simulink model "e4_tank_reactor_no_error_dyn"  (R2020a)
settings: Solver=FixedStepAuto  StartTime=0.0  StopTime=options.T_train  FixedStep=options.dt  RelTol=1e-3
PreLoadFcn:
  | load e4_PIDGainSchedExample.mat
model workspace (MAT data in the model file):
  op_snapshot1 : handle (value not decoded)
values from neighbouring files (symbols this model uses):
  C = [2 3 4 5 6 7 8 9]    [e4_PIDGainSchedExample.mat]
undefined symbols (not defined in the file or in its folder): Controllers, D, I, N, options, P, sigbuilder_block
libraries: neural x132, simulink x2, simulink_need_slupdate x1
(part 4 of 6)

== system e4_tank_reactor_no_error_dyn/NN/Layer 3/Delays 1 ==
  "p{3}" : Inport  PortDimensions=30
      mask Display: e = 0.06;c1 = [120 230 180]/255;c2 = ([120 230 180]+0)/(256+128);c3 = ([120 230 180]+128)/(256+128);patch([0 1 1 0],[0 0 1 1],c1);patch([0 1 1 1-e 1-e 0+e],[0 0 1 1-e 0+e 0+e],c2);patch([0 0 1 1-e 0+e 0+e],[0 1 1 1-e 1-e 0+e],c3);plot([0 1 1 0 0],[0 0 1 1 0]);
  mux : Mux  Inputs=1
      mask Display: e = 0.06;c1 = [120 150 230]/255;c2 = ([120 150 230]+0)/383;c3 = ([120 150 230]+128)/383;patch([0 1 1 0],[0 0 1 1],c1);patch([0 1 1 1-e 1-e 0+e],[0 0 1 1-e 0+e 0+e],c2);patch([0 0 1 1-e 0+e 0+e],[0 1 1 1-e 1-e 0+e],c3);plot([0 1 1 0 0],[0 0 1 1 0]);disp('Mux')
  "pd{3,2}" : Outport
      mask Display: e = 0.06;c1 = [120 230 180]/255;c2 = ([120 230 180]+0)/(256+128);c3 = ([120 230 180]+128)/(256+128);patch([0 1 1 0],[0 0 1 1],c1);patch([0 1 1 1-e 1-e 0+e],[0 0 1 1-e 0+e 0+e],c2);patch([0 0 1 1-e 0+e 0+e],[0 1 1 1-e 1-e 0+e],c3);plot([0 1 1 0 0],[0 0 1 1 0]);
  wires:
  "p{3}"/1 -> mux/1
  mux/1 -> "pd{3,2}"/1

== system e4_tank_reactor_no_error_dyn/NN/Layer 3/LW{3,2} ==
  "ad{3,2}" : Inport  PortDimensions=30
      mask Display: e = 0.06;c1 = [120 230 180]/255;c2 = ([120 230 180]+0)/(256+128);c3 = ([120 230 180]+128)/(256+128);patch([0 1 1 0],[0 0 1 1],c1);patch([0 1 1 1-e 1-e 0+e],[0 0 1 1-e 0+e 0+e],c2);patch([0 0 1 1-e 0+e 0+e],[0 1 1 1-e 1-e 0+e],c3);plot([0 1 1 0 0],[0 0 1 1 0]);
  "IW{3,2}(1,:)'" : Constant  Value=[-0.0464803788192958700076218292451812885701656341552734375;-0.22366786030205820789973358841962181031703948974609375;0.09453253511773705708431947414283058606088161468505859375;0.303300315972412859455431544120074249804019927978515625;-0.001379384046064999029546083164632364059798419475555419921875;-0.11257074515520755497721694382562418468296527862548828125;-0.10240733375565913565452547118184156715869903564453125;0.05926219251905744112018936675667646341025829315185546875;-0.1213117218938437880115799316627089865505695343017578125;-0.07223384242120071963011440629998105578124523162841796875;-0.08011048819587056335489450020759250037372112274169921875;-0.01346694101269302508427916365008059074170887470245361328125;-0.0161980791466645283882552774912255699746310710906982421875;-0.13100020285189517554869098603376187384128570556640625;-0.325236116042997736030883970670402050018310546875;-0.016627521139407630546003247218322940170764923095703125;0.01071971917916101670054107586338432156480848789215087890625;-0.00444701838994284413819624290908905095420777797698974609375;0.066701814396379177640739044363726861774921417236328125;0.097044878239975762568292338983155786991119384765625;-0.24982480627273417894684826023876667022705078125;-0.0259297241783282804428178991429376765154302120208740234375;0.176353365166070863434555349158472381532192230224609375;-0.0778415585458839542898346053334535099565982818603515625;0.28946783805742037909425334873958490788936614990234375;-0.0264164360665425819452156730449132737703621387481689453125;0.039973819515048851502836413374097901396453380584716796875;0.08025452129389230859768389336750260554254055023193359375;0.4427935738953550082186438885401003062725067138671875;-0.344840403191533029225723794297664426267147064208984375]
      mask Display: e = 0.06;c1 = [120 150 230]/255;c2 = ([120 150 230]+0)/383;c3 = ([120 150 230]+128)/383;patch([0 1 1 0],[0 0 1 1],c1);patch([0 1 1 1-e 1-e 0+e],[0 0 1 1-e 0+e 0+e],c2);patch([0 0 1 1-e 0+e 0+e],[0 1 1 1-e 1-e 0+e],c3);plot([0 1 1 0 0],[0 0 1 1 0]);disp('weights');
  Mux : Mux  Inputs=1
      mask Display: e = 0.06;c1 = [120 150 230]/255;c2 = ([120 150 230]+0)/383;c3 = ([120 150 230]+128)/383;patch([0 1 1 0],[0 0 1 1],c1);patch([0 1 1 1-e 1-e 0+e],[0 0 1 1-e 0+e 0+e],c2);patch([0 0 1 1-e 0+e 0+e],[0 1 1 1-e 1-e 0+e],c3);plot([0 1 1 0 0],[0 0 1 1 0]);disp('Mux');
  dotprod1 : neural/Weight Functions/dotprod
  "lz{3,2}" : Outport
      mask Display: e = 0.06;c1 = [120 230 180]/255;c2 = ([120 230 180]+0)/(256+128);c3 = ([120 230 180]+128)/(256+128);patch([0 1 1 0],[0 0 1 1],c1);patch([0 1 1 1-e 1-e 0+e],[0 0 1 1-e 0+e 0+e],c2);patch([0 0 1 1-e 0+e 0+e],[0 1 1 1-e 1-e 0+e],c3);plot([0 1 1 0 0],[0 0 1 1 0]);
  wires:
  "IW{3,2}(1,:)'"/1 -> dotprod1/1
  "ad{3,2}"/1 -> dotprod1/2
  dotprod1/1 -> Mux/1
  Mux/1 -> "lz{3,2}"/1

== system e4_tank_reactor_no_error_dyn/NN_cex_1/Layer 1/Delays 1 ==
  "p{1}" : Inport  PortDimensions=8
      mask Display: e = 0.06;c1 = [120 230 180]/255;c2 = ([120 230 180]+0)/(256+128);c3 = ([120 230 180]+128)/(256+128);patch([0 1 1 0],[0 0 1 1],c1);patch([0 1 1 1-e 1-e 0+e],[0 0 1 1-e 0+e 0+e],c2);patch([0 0 1 1-e 0+e 0+e],[0 1 1 1-e 1-e 0+e],c3);plot([0 1 1 0 0],[0 0 1 1 0]);
  mux : Mux  Inputs=1
      mask Display: e = 0.06;c1 = [120 150 230]/255;c2 = ([120 150 230]+0)/383;c3 = ([120 150 230]+128)/383;patch([0 1 1 0],[0 0 1 1],c1);patch([0 1 1 1-e 1-e 0+e],[0 0 1 1-e 0+e 0+e],c2);patch([0 0 1 1-e 0+e 0+e],[0 1 1 1-e 1-e 0+e],c3);plot([0 1 1 0 0],[0 0 1 1 0]);disp('Mux')
  "pd{1,1}" : Outport
      mask Display: e = 0.06;c1 = [120 230 180]/255;c2 = ([120 230 180]+0)/(256+128);c3 = ([120 230 180]+128)/(256+128);patch([0 1 1 0],[0 0 1 1],c1);patch([0 1 1 1-e 1-e 0+e],[0 0 1 1-e 0+e 0+e],c2);patch([0 0 1 1-e 0+e 0+e],[0 1 1 1-e 1-e 0+e],c3);plot([0 1 1 0 0],[0 0 1 1 0]);
  wires:
  "p{1}"/1 -> mux/1
  mux/1 -> "pd{1,1}"/1

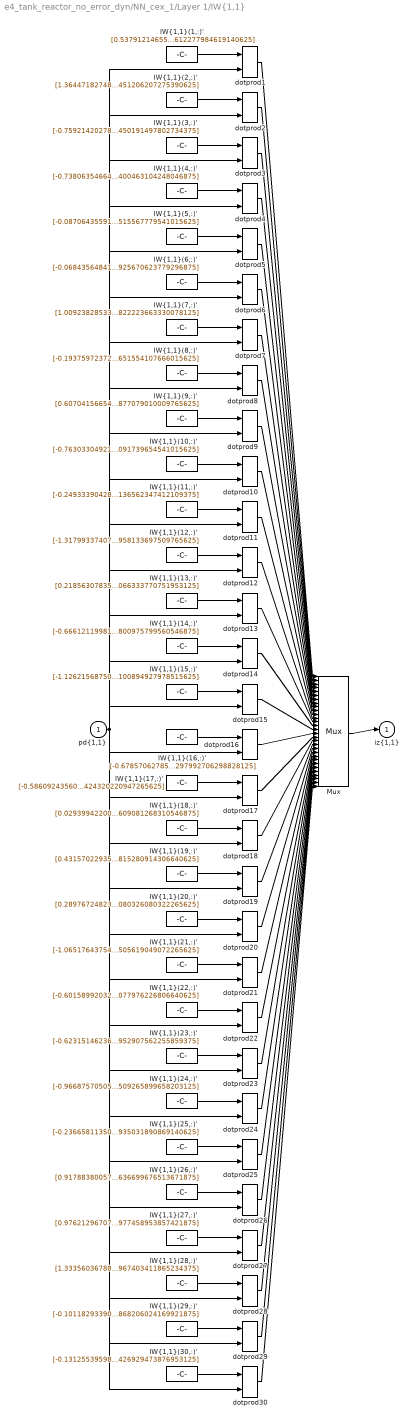
== system e4_tank_reactor_no_error_dyn/NN_cex_1/Layer 1/IW{1,1} ==
  "pd{1,1}" : Inport  PortDimensions=8
      mask Display: e = 0.06;c1 = [120 230 180]/255;c2 = ([120 230 180]+0)/(256+128);c3 = ([120 230 180]+128)/(256+128);patch([0 1 1 0],[0 0 1 1],c1);patch([0 1 1 1-e 1-e 0+e],[0 0 1 1-e 0+e 0+e],c2);patch([0 0 1 1-e 0+e 0+e],[0 1 1 1-e 1-e 0+e],c3);plot([0 1 1 0 0],[0 0 1 1 0]);
  "IW{1,1}(1,:)'" : Constant  Value=[0.5379121465548728497907404744182713329792022705078125;-0.4891956453284975747664020673255436122417449951171875;0.453842574705631829345975347678177058696746826171875;-2.25657579421494514093637917540036141872406005859375;-0.2491786341732944720650522185678710229694843292236328125;-0.1742315599251909319367115358545561321079730987548828125;-1.8134520137386844762517057461082004010677337646484375;-0.86465480796345206560005181017913855612277984619140625]
      mask Display: e = 0.06;c1 = [120 150 230]/255;c2 = ([120 150 230]+0)/383;c3 = ([120 150 230]+128)/383;patch([0 1 1 0],[0 0 1 1],c1);patch([0 1 1 1-e 1-e 0+e],[0 0 1 1-e 0+e 0+e],c2);patch([0 0 1 1-e 0+e 0+e],[0 1 1 1-e 1-e 0+e],c3);plot([0 1 1 0 0],[0 0 1 1 0]);disp('Weights');
  "IW{1,1}(10,:)'" : Constant  Value=[-0.7630330492125356744992359381285496056079864501953125;-0.1535957203894409150990441048634238541126251220703125;-1.1348681599380225915041364714852534234523773193359375;1.1072262797523821920009368113824166357517242431640625;-0.5333903505207240325347584075643680989742279052734375;-0.51407599439698958843081300074118189513683319091796875;1.1142771208274837579921268115867860615253448486328125;-1.5225707798856602526171855060965754091739654541015625]
      mask Display: e = 0.06;c1 = [120 150 230]/255;c2 = ([120 150 230]+0)/383;c3 = ([120 150 230]+128)/383;patch([0 1 1 0],[0 0 1 1],c1);patch([0 1 1 1-e 1-e 0+e],[0 0 1 1-e 0+e 0+e],c2);patch([0 0 1 1-e 0+e 0+e],[0 1 1 1-e 1-e 0+e],c3);plot([0 1 1 0 0],[0 0 1 1 0]);disp('Weights');
  "IW{1,1}(11,:)'" : Constant  Value=[-0.2493339042877996403202445208080462180078029632568359375;-0.044937110292640324027413356589022441767156124114990234375;-0.89629168879976617301252872493932954967021942138671875;-0.94562916108070871334945195485488511621952056884765625;1.1876936211677457944091429453692398965358734130859375;-0.54144662550112754306752549382508732378482818603515625;1.0278469665745559868952341275871731340885162353515625;-0.47008241850572252129580874679959379136562347412109375]
      mask Display: e = 0.06;c1 = [120 150 230]/255;c2 = ([120 150 230]+0)/383;c3 = ([120 150 230]+128)/383;patch([0 1 1 0],[0 0 1 1],c1);patch([0 1 1 1-e 1-e 0+e],[0 0 1 1-e 0+e 0+e],c2);patch([0 0 1 1-e 0+e 0+e],[0 1 1 1-e 1-e 0+e],c3);plot([0 1 1 0 0],[0 0 1 1 0]);disp('Weights');
  "IW{1,1}(12,:)'" : Constant  Value=[-1.31799337407540662070459802635014057159423828125;1.08939525062658759679834474809467792510986328125;1.100424298584484983365427979151718318462371826171875;-0.35666979575481694286764877688256092369556427001953125;0.293602012746428442380164369751582853496074676513671875;0.98047102923849960287583371609798632562160491943359375;-0.4527363536410680122656913226819597184658050537109375;0.78261151530452244262647809591726399958133697509765625]
      mask Display: e = 0.06;c1 = [120 150 230]/255;c2 = ([120 150 230]+0)/383;c3 = ([120 150 230]+128)/383;patch([0 1 1 0],[0 0 1 1],c1);patch([0 1 1 1-e 1-e 0+e],[0 0 1 1-e 0+e 0+e],c2);patch([0 0 1 1-e 0+e 0+e],[0 1 1 1-e 1-e 0+e],c3);plot([0 1 1 0 0],[0 0 1 1 0]);disp('Weights');
  "IW{1,1}(13,:)'" : Constant  Value=[0.2185630783525124576360809669495210982859134674072265625;1.153492150410983629882366585661657154560089111328125;-0.281741742390723970412835797105799429118633270263671875;0.430450607409247065771040752224507741630077362060546875;-0.2156642293311239744202367774050799198448657989501953125;-1.28844042664953928323257059673778712749481201171875;0.226045890241030555944945490409736521542072296142578125;0.81490911166711743618407126632519066333770751953125]
      mask Display: e = 0.06;c1 = [120 150 230]/255;c2 = ([120 150 230]+0)/383;c3 = ([120 150 230]+128)/383;patch([0 1 1 0],[0 0 1 1],c1);patch([0 1 1 1-e 1-e 0+e],[0 0 1 1-e 0+e 0+e],c2);patch([0 0 1 1-e 0+e 0+e],[0 1 1 1-e 1-e 0+e],c3);plot([0 1 1 0 0],[0 0 1 1 0]);disp('Weights');
  "IW{1,1}(14,:)'" : Constant  Value=[-0.66612119981264938939347075574914924800395965576171875;0.70433163322524794391910063495743088424205780029296875;1.51350451798926766144859357154928147792816162109375;0.135062226669892371244685591591405682265758514404296875;-0.6139892191890223838157680802396498620510101318359375;0.785352351475125498581064675818197429180145263671875;0.2797159376970330679768039772170595824718475341796875;2.02825949533217197995327296666800975799560546875]
      mask Display: e = 0.06;c1 = [120 150 230]/255;c2 = ([120 150 230]+0)/383;c3 = ([120 150 230]+128)/383;patch([0 1 1 0],[0 0 1 1],c1);patch([0 1 1 1-e 1-e 0+e],[0 0 1 1-e 0+e 0+e],c2);patch([0 0 1 1-e 0+e 0+e],[0 1 1 1-e 1-e 0+e],c3);plot([0 1 1 0 0],[0 0 1 1 0]);disp('Weights');
  "IW{1,1}(15,:)'" : Constant  Value=[-1.126215687500734308201799649395979940891265869140625;0.5324020585546609396487838239409029483795166015625;0.275269474209976883205541753341094590723514556884765625;0.9901222314779591915367973342654295265674591064453125;-0.8749086639717464919385747634805738925933837890625;0.38958898768835348302985721602453850209712982177734375;-0.073311773987459749601924841044819913804531097412109375;0.84648532346684801641600870425463654100894927978515625]
      mask Display: e = 0.06;c1 = [120 150 230]/255;c2 = ([120 150 230]+0)/383;c3 = ([120 150 230]+128)/383;patch([0 1 1 0],[0 0 1 1],c1);patch([0 1 1 1-e 1-e 0+e],[0 0 1 1-e 0+e 0+e],c2);patch([0 0 1 1-e 0+e 0+e],[0 1 1 1-e 1-e 0+e],c3);plot([0 1 1 0 0],[0 0 1 1 0]);disp('Weights');
  "IW{1,1}(16,:)'" : Constant  Value=[-0.6785706278511709488299175063730217516422271728515625;-1.1815839277690927122677067018230445683002471923828125;-0.70641636384911199453284780247486196458339691162109375;1.0070190226252275778051625820808112621307373046875;0.0220071147234353892141456299214041791856288909912109375;0.0942288635999547763422157231616438366472721099853515625;0.9300673100145997462817604173324070870876312255859375;1.23984567310700288800262569566257297992706298828125]
      mask Display: e = 0.06;c1 = [120 150 230]/255;c2 = ([120 150 230]+0)/383;c3 = ([120 150 230]+128)/383;patch([0 1 1 0],[0 0 1 1],c1);patch([0 1 1 1-e 1-e 0+e],[0 0 1 1-e 0+e 0+e],c2);patch([0 0 1 1-e 0+e 0+e],[0 1 1 1-e 1-e 0+e],c3);plot([0 1 1 0 0],[0 0 1 1 0]);disp('Weights');
  "IW{1,1}(17,:)'" : Constant  Value=[-0.5860924356005476898445749611710198223590850830078125;0.851474377071834709340691915713250637054443359375;-0.1567050173144934610558465237772907130420207977294921875;-0.68500297234766527321170315190101973712444305419921875;0.8118387502084571938354429221362806856632232666015625;-1.154822097518132917315369923016987740993499755859375;0.60957063637892872076662342806230299174785614013671875;0.375224662295090161112653959207818843424320220947265625]
      mask Display: e = 0.06;c1 = [120 150 230]/255;c2 = ([120 150 230]+0)/383;c3 = ([120 150 230]+128)/383;patch([0 1 1 0],[0 0 1 1],c1);patch([0 1 1 1-e 1-e 0+e],[0 0 1 1-e 0+e 0+e],c2);patch([0 0 1 1-e 0+e 0+e],[0 1 1 1-e 1-e 0+e],c3);plot([0 1 1 0 0],[0 0 1 1 0]);disp('Weights');
  "IW{1,1}(18,:)'" : Constant  Value=[0.02939942200266887351034483799594454467296600341796875;-0.299792566816287131548079969434184022247791290283203125;-0.60369148945598005706614230803097598254680633544921875;-0.13551079379416908210487235919572412967681884765625;0.419757903271528010069602032672264613211154937744140625;0.799628628682101716407260028063319623470306396484375;0.5142029788862163552920492293196730315685272216796875;-0.223354218656821312816163072056951932609081268310546875]
      mask Display: e = 0.06;c1 = [120 150 230]/255;c2 = ([120 150 230]+0)/383;c3 = ([120 150 230]+128)/383;patch([0 1 1 0],[0 0 1 1],c1);patch([0 1 1 1-e 1-e 0+e],[0 0 1 1-e 0+e 0+e],c2);patch([0 0 1 1-e 0+e 0+e],[0 1 1 1-e 1-e 0+e],c3);plot([0 1 1 0 0],[0 0 1 1 0]);disp('Weights');
  "IW{1,1}(19,:)'" : Constant  Value=[0.431570229354902357155054914983338676393032073974609375;0.3345690055866470391521261262823827564716339111328125;1.0469583717854737958674604669795371592044830322265625;0.72253391100106190148011364726698957383632659912109375;-0.545424201225733984443877488956786692142486572265625;0.0101024782301144915030999271721157128922641277313232421875;-0.167124150696403350746521709879743866622447967529296875;-1.454795311551409842110160752781666815280914306640625]
      mask Display: e = 0.06;c1 = [120 150 230]/255;c2 = ([120 150 230]+0)/383;c3 = ([120 150 230]+128)/383;patch([0 1 1 0],[0 0 1 1],c1);patch([0 1 1 1-e 1-e 0+e],[0 0 1 1-e 0+e 0+e],c2);patch([0 0 1 1-e 0+e 0+e],[0 1 1 1-e 1-e 0+e],c3);plot([0 1 1 0 0],[0 0 1 1 0]);disp('Weights');
  "IW{1,1}(2,:)'" : Constant  Value=[1.3644718274849083616828693266143091022968292236328125;-0.6113012571242200099419505932019092142581939697265625;0.219308348802042252234656416476354934275150299072265625;-0.050551389902864729553044753629365004599094390869140625;1.1572125475706760422411889521754346787929534912109375;0.364957647871666068795093451626598834991455078125;1.3711534269785918827011528264847584068775177001953125;-0.634282382592994853354184670024551451206207275390625]
      mask Display: e = 0.06;c1 = [120 150 230]/255;c2 = ([120 150 230]+0)/383;c3 = ([120 150 230]+128)/383;patch([0 1 1 0],[0 0 1 1],c1);patch([0 1 1 1-e 1-e 0+e],[0 0 1 1-e 0+e 0+e],c2);patch([0 0 1 1-e 0+e 0+e],[0 1 1 1-e 1-e 0+e],c3);plot([0 1 1 0 0],[0 0 1 1 0]);disp('Weights');
  "IW{1,1}(20,:)'" : Constant  Value=[0.289767248236110164238965580807416699826717376708984375;-1.6550121300658424683405200994457118213176727294921875;0.66498678015265133556255250368849374353885650634765625;-0.358201489276206597178742185860755853354930877685546875;1.2038940893287257694055369938723742961883544921875;-0.7811727388937643734578841758775524795055389404296875;-0.293491754609760124861139729546266607940196990966796875;-0.87310715343854161663017521277652122080326080322265625]
      mask Display: e = 0.06;c1 = [120 150 230]/255;c2 = ([120 150 230]+0)/383;c3 = ([120 150 230]+128)/383;patch([0 1 1 0],[0 0 1 1],c1);patch([0 1 1 1-e 1-e 0+e],[0 0 1 1-e 0+e 0+e],c2);patch([0 0 1 1-e 0+e 0+e],[0 1 1 1-e 1-e 0+e],c3);plot([0 1 1 0 0],[0 0 1 1 0]);disp('Weights');
  "IW{1,1}(21,:)'" : Constant  Value=[-1.0651764375415757601928135045454837381839752197265625;-0.05093105960695791523118458599128643982112407684326171875;0.10166969326193157907578523690972360782325267791748046875;0.787265018557109730323873009183444082736968994140625;-1.0383486929548138011369928790372796356678009033203125;1.0418870137961391275638334263931028544902801513671875;-2.059969041537390577190080875880084931850433349609375;-0.363346918231178594993480146513320505619049072265625]
      mask Display: e = 0.06;c1 = [120 150 230]/255;c2 = ([120 150 230]+0)/383;c3 = ([120 150 230]+128)/383;patch([0 1 1 0],[0 0 1 1],c1);patch([0 1 1 1-e 1-e 0+e],[0 0 1 1-e 0+e 0+e],c2);patch([0 0 1 1-e 0+e 0+e],[0 1 1 1-e 1-e 0+e],c3);plot([0 1 1 0 0],[0 0 1 1 0]);disp('Weights');
  "IW{1,1}(22,:)'" : Constant  Value=[-0.60158992032533775695668509797542355954647064208984375;-1.3680290127964724877784874479402787983417510986328125;-0.87834865591767175008186541163013316690921783447265625;-0.2207869194855082983774963167888927273452281951904296875;-0.11766408992345871176166127725082333199679851531982421875;0.97286536737283990650126952459686435759067535400390625;-0.76589398294444854808915579269523732364177703857421875;-0.449268913356635213318668320425786077976226806640625]
      mask Display: e = 0.06;c1 = [120 150 230]/255;c2 = ([120 150 230]+0)/383;c3 = ([120 150 230]+128)/383;patch([0 1 1 0],[0 0 1 1],c1);patch([0 1 1 1-e 1-e 0+e],[0 0 1 1-e 0+e 0+e],c2);patch([0 0 1 1-e 0+e 0+e],[0 1 1 1-e 1-e 0+e],c3);plot([0 1 1 0 0],[0 0 1 1 0]);disp('Weights');
  "IW{1,1}(23,:)'" : Constant  Value=[-0.62315146236465379647739837309927679598331451416015625;0.700611887631571672585550913936458528041839599609375;-1.253865587185787777713130708434619009494781494140625;0.12191954613290224840316255949801416136324405670166015625;0.02485690435094556338668780881562270224094390869140625;-0.97564300724903951778088639912311919033527374267578125;-1.3728328336670490017468182486481964588165283203125;-0.476364886346988425369630704153678379952907562255859375]
      mask Display: e = 0.06;c1 = [120 150 230]/255;c2 = ([120 150 230]+0)/383;c3 = ([120 150 230]+128)/383;patch([0 1 1 0],[0 0 1 1],c1);patch([0 1 1 1-e 1-e 0+e],[0 0 1 1-e 0+e 0+e],c2);patch([0 0 1 1-e 0+e 0+e],[0 1 1 1-e 1-e 0+e],c3);plot([0 1 1 0 0],[0 0 1 1 0]);disp('Weights');
  "IW{1,1}(24,:)'" : Constant  Value=[-0.9668757050519467544091867239330895245075225830078125;1.8074949802424502554032414991525001823902130126953125;0.1509264792134751009822224432355142198503017425537109375;0.56079147047206401310859291697852313518524169921875;-0.86686870292866513576512943473062478005886077880859375;0.00566384031475077563688724779922267771326005458831787109375;-0.5858846977314049464524714494473300874233245849609375;-0.35202968611922369479572125783306546509265899658203125]
      mask Display: e = 0.06;c1 = [120 150 230]/255;c2 = ([120 150 230]+0)/383;c3 = ([120 150 230]+128)/383;patch([0 1 1 0],[0 0 1 1],c1);patch([0 1 1 1-e 1-e 0+e],[0 0 1 1-e 0+e 0+e],c2);patch([0 0 1 1-e 0+e 0+e],[0 1 1 1-e 1-e 0+e],c3);plot([0 1 1 0 0],[0 0 1 1 0]);disp('Weights');
  "IW{1,1}(25,:)'" : Constant  Value=[-0.2366581135092546139819802419879124499857425689697265625;-1.1565509789181909194866193502093665301799774169921875;0.356085223857672328318102472621831111609935760498046875;0.51409424697715355723204311289009638130664825439453125;-0.73596497723560927450847657382837496697902679443359375;0.2926871688236143409511669233324937522411346435546875;-1.3190253126527398119804956877487711608409881591796875;1.3400461156173195664820241290726698935031890869140625]
      mask Display: e = 0.06;c1 = [120 150 230]/255;c2 = ([120 150 230]+0)/383;c3 = ([120 150 230]+128)/383;patch([0 1 1 0],[0 0 1 1],c1);patch([0 1 1 1-e 1-e 0+e],[0 0 1 1-e 0+e 0+e],c2);patch([0 0 1 1-e 0+e 0+e],[0 1 1 1-e 1-e 0+e],c3);plot([0 1 1 0 0],[0 0 1 1 0]);disp('Weights');
  "IW{1,1}(26,:)'" : Constant  Value=[0.91788380057172869186388197704218327999114990234375;1.15538220933264046408339709159918129444122314453125;0.8339026184910924843762813907233066856861114501953125;0.36652474061263762283857658985652960836887359619140625;-0.038492407008773772691956338576346752233803272247314453125;0.10236621810067032811719656137938727624714374542236328125;0.6540196398808897360055425451719202101230621337890625;0.3290186601830498158705040623317472636699676513671875]
      mask Display: e = 0.06;c1 = [120 150 230]/255;c2 = ([120 150 230]+0)/383;c3 = ([120 150 230]+128)/383;patch([0 1 1 0],[0 0 1 1],c1);patch([0 1 1 1-e 1-e 0+e],[0 0 1 1-e 0+e 0+e],c2);patch([0 0 1 1-e 0+e 0+e],[0 1 1 1-e 1-e 0+e],c3);plot([0 1 1 0 0],[0 0 1 1 0]);disp('Weights');
  "IW{1,1}(27,:)'" : Constant  Value=[0.9762129670729109420790337026119232177734375;-0.66682266891450880930136690949439071118831634521484375;0.14765647832353767654467446845956146717071533203125;-0.744789681230276556789249298162758350372314453125;0.664196844738051073164797344361431896686553955078125;0.74611195556748632906618468041415326297283172607421875;0.796280949331405363267322172760032117366790771484375;-0.1026615824494294393343096771786804310977458953857421875]
      mask Display: e = 0.06;c1 = [120 150 230]/255;c2 = ([120 150 230]+0)/383;c3 = ([120 150 230]+128)/383;patch([0 1 1 0],[0 0 1 1],c1);patch([0 1 1 1-e 1-e 0+e],[0 0 1 1-e 0+e 0+e],c2);patch([0 0 1 1-e 0+e 0+e],[0 1 1 1-e 1-e 0+e],c3);plot([0 1 1 0 0],[0 0 1 1 0]);disp('Weights');
  "IW{1,1}(28,:)'" : Constant  Value=[1.33356036788779430679596771369688212871551513671875;0.2356965321398985790946056795291951857507228851318359375;-0.232455208957773551414760504485457204282283782958984375;-0.178559020015909786227581435014144517481327056884765625;0.89276443639134417384894959468510933220386505126953125;-0.7558328227887614048086106777191162109375;0.1388690330901915237493682298008934594690799713134765625;1.4965266154135272724801097865565679967403411865234375]
      mask Display: e = 0.06;c1 = [120 150 230]/255;c2 = ([120 150 230]+0)/383;c3 = ([120 150 230]+128)/383;patch([0 1 1 0],[0 0 1 1],c1);patch([0 1 1 1-e 1-e 0+e],[0 0 1 1-e 0+e 0+e],c2);patch([0 0 1 1-e 0+e 0+e],[0 1 1 1-e 1-e 0+e],c3);plot([0 1 1 0 0],[0 0 1 1 0]);disp('Weights');
  "IW{1,1}(29,:)'" : Constant  Value=[-0.10118293390951231536245558118025655858218669891357421875;0.06434138355125963715241965701352455653250217437744140625;-0.69739459415743121351027866694494150578975677490234375;0.79226095210926195111511560753569938242435455322265625;-0.90436354784671169060317197363474406301975250244140625;-1.23209955543295990310070919804275035858154296875;1.092697805682678602323676386731676757335662841796875;0.4849451497525627541307358114863745868206024169921875]
      mask Display: e = 0.06;c1 = [120 150 230]/255;c2 = ([120 150 230]+0)/383;c3 = ([120 150 230]+128)/383;patch([0 1 1 0],[0 0 1 1],c1);patch([0 1 1 1-e 1-e 0+e],[0 0 1 1-e 0+e 0+e],c2);patch([0 0 1 1-e 0+e 0+e],[0 1 1 1-e 1-e 0+e],c3);plot([0 1 1 0 0],[0 0 1 1 0]);disp('Weights');
  "IW{1,1}(3,:)'" : Constant  Value=[-0.75921420278456952512868838311987929046154022216796875;1.1246289809493703604204029034008271992206573486328125;0.357400133672493292014138432932668365538120269775390625;-1.2713477569867224215016676680534146726131439208984375;0.79391674854068738920176429019193165004253387451171875;0.71648590916453891441761925307218916714191436767578125;0.359501923755549401828801592273521237075328826904296875;0.44836330481205288744916970244958065450191497802734375]
      mask Display: e = 0.06;c1 = [120 150 230]/255;c2 = ([120 150 230]+0)/383;c3 = ([120 150 230]+128)/383;patch([0 1 1 0],[0 0 1 1],c1);patch([0 1 1 1-e 1-e 0+e],[0 0 1 1-e 0+e 0+e],c2);patch([0 0 1 1-e 0+e 0+e],[0 1 1 1-e 1-e 0+e],c3);plot([0 1 1 0 0],[0 0 1 1 0]);disp('Weights');
  "IW{1,1}(30,:)'" : Constant  Value=[-0.13125539598877633551410326617769896984100341796875;-1.369496947258934227420468232594430446624755859375;-1.236078110166821009130444508627988398075103759765625;-0.72204748831942466846811612413148395717144012451171875;0.761983709141599963032831510645337402820587158203125;0.90521509240511310867560723636415787041187286376953125;-0.610208060498799387261215088074095547199249267578125;-0.78955110194053024219584813181427307426929473876953125]
      mask Display: e = 0.06;c1 = [120 150 230]/255;c2 = ([120 150 230]+0)/383;c3 = ([120 150 230]+128)/383;patch([0 1 1 0],[0 0 1 1],c1);patch([0 1 1 1-e 1-e 0+e],[0 0 1 1-e 0+e 0+e],c2);patch([0 0 1 1-e 0+e 0+e],[0 1 1 1-e 1-e 0+e],c3);plot([0 1 1 0 0],[0 0 1 1 0]);disp('Weights');
  "IW{1,1}(4,:)'" : Constant  Value=[-0.73806354664510143148703491533524356782436370849609375;-1.685791217549649001483658139477483928203582763671875;0.34882725222296262490573326431331224739551544189453125;-0.736035017934379087733987034880556166172027587890625;0.44053466594436374581533755190321244299411773681640625;0.412365071467659161097429887377074919641017913818359375;-0.2378886841219116921042342482905951328575611114501953125;0.7315009545194779416732444587978534400463104248046875]
      mask Display: e = 0.06;c1 = [120 150 230]/255;c2 = ([120 150 230]+0)/383;c3 = ([120 150 230]+128)/383;patch([0 1 1 0],[0 0 1 1],c1);patch([0 1 1 1-e 1-e 0+e],[0 0 1 1-e 0+e 0+e],c2);patch([0 0 1 1-e 0+e 0+e],[0 1 1 1-e 1-e 0+e],c3);plot([0 1 1 0 0],[0 0 1 1 0]);disp('Weights');
  "IW{1,1}(5,:)'" : Constant  Value=[-0.087064355913521851437764098591287620365619659423828125;-0.69226769568504764595928691051085479557514190673828125;-0.052166682908634430526628733559846295975148677825927734375;-1.78817229179241365955022047273814678192138671875;-0.202354836069230825668086026780656538903713226318359375;0.424849282091239732750409530126489698886871337890625;0.135767011506318480140720339477411471307277679443359375;0.80800721671806796653214632897288538515567779541015625]
      mask Display: e = 0.06;c1 = [120 150 230]/255;c2 = ([120 150 230]+0)/383;c3 = ([120 150 230]+128)/383;patch([0 1 1 0],[0 0 1 1],c1);patch([0 1 1 1-e 1-e 0+e],[0 0 1 1-e 0+e 0+e],c2);patch([0 0 1 1-e 0+e 0+e],[0 1 1 1-e 1-e 0+e],c3);plot([0 1 1 0 0],[0 0 1 1 0]);disp('Weights');
  "IW{1,1}(6,:)'" : Constant  Value=[-0.068435648417951522315405554763856343924999237060546875;0.470302497384609774488950506565743125975131988525390625;-0.94847648407455376062813456883304752409458160400390625;-0.726406908026099973341160875861532986164093017578125;-1.0497552281827309261785785565734840929508209228515625;-0.77473558474632919779168105378630571067333221435546875;-0.00533671882829562203853779323026174097321927547454833984375;-0.46811053703059346542403318380820564925670623779296875]
      mask Display: e = 0.06;c1 = [120 150 230]/255;c2 = ([120 150 230]+0)/383;c3 = ([120 150 230]+128)/383;patch([0 1 1 0],[0 0 1 1],c1);patch([0 1 1 1-e 1-e 0+e],[0 0 1 1-e 0+e 0+e],c2);patch([0 0 1 1-e 0+e 0+e],[0 1 1 1-e 1-e 0+e],c3);plot([0 1 1 0 0],[0 0 1 1 0]);disp('Weights');
  "IW{1,1}(7,:)'" : Constant  Value=[1.0092382853340426951405106592574156820774078369140625;-1.139950344657586267516080624773167073726654052734375;-0.62773609805279562134927573424647562205791473388671875;-0.057749342132758528511882190059623098932206630706787109375;1.065565365614550064066179402288980782032012939453125;1.931400163213802922967943231924436986446380615234375;0.9316086738097215658171990071423351764678955078125;-0.8470511738152186609340787981636822223663330078125]
      mask Display: e = 0.06;c1 = [120 150 230]/255;c2 = ([120 150 230]+0)/383;c3 = ([120 150 230]+128)/383;patch([0 1 1 0],[0 0 1 1],c1);patch([0 1 1 1-e 1-e 0+e],[0 0 1 1-e 0+e 0+e],c2);patch([0 0 1 1-e 0+e 0+e],[0 1 1 1-e 1-e 0+e],c3);plot([0 1 1 0 0],[0 0 1 1 0]);disp('Weights');
  "IW{1,1}(8,:)'" : Constant  Value=[-0.193759723728735178127635663258843123912811279296875;-0.320358020393277376225427133249468170106410980224609375;0.54372272546971800455395396056701429188251495361328125;0.307262692964356098901390623723273165524005889892578125;-0.9551945943378965520054180160514079034328460693359375;-0.1880539563659444912691043327868101187050342559814453125;0.93005272750526823966055189885082654654979705810546875;-1.267124174526627289338875925750471651554107666015625]
      mask Display: e = 0.06;c1 = [120 150 230]/255;c2 = ([120 150 230]+0)/383;c3 = ([120 150 230]+128)/383;patch([0 1 1 0],[0 0 1 1],c1);patch([0 1 1 1-e 1-e 0+e],[0 0 1 1-e 0+e 0+e],c2);patch([0 0 1 1-e 0+e 0+e],[0 1 1 1-e 1-e 0+e],c3);plot([0 1 1 0 0],[0 0 1 1 0]);disp('Weights');
  "IW{1,1}(9,:)'" : Constant  Value=[0.60704156654122332081868762543308548629283905029296875;0.9994649923571865546279013869934715330600738525390625;-1.8269672307963611412873206063522957265377044677734375;-0.6494087026862265243920546708977781236171722412109375;-1.1806609578532907267600648992811329662799835205078125;1.51802367372904001285860431380569934844970703125;0.454130230801493783854283492473769001662731170654296875;-1.092844909786183649202939704991877079010009765625]
      mask Display: e = 0.06;c1 = [120 150 230]/255;c2 = ([120 150 230]+0)/383;c3 = ([120 150 230]+128)/383;patch([0 1 1 0],[0 0 1 1],c1);patch([0 1 1 1-e 1-e 0+e],[0 0 1 1-e 0+e 0+e],c2);patch([0 0 1 1-e 0+e 0+e],[0 1 1 1-e 1-e 0+e],c3);plot([0 1 1 0 0],[0 0 1 1 0]);disp('Weights');
  Mux : Mux  Inputs=30
      mask Display: e = 0.06;c1 = [120 150 230]/255;c2 = ([120 150 230]+0)/383;c3 = ([120 150 230]+128)/383;patch([0 1 1 0],[0 0 1 1],c1);patch([0 1 1 1-e 1-e 0+e],[0 0 1 1-e 0+e 0+e],c2);patch([0 0 1 1-e 0+e 0+e],[0 1 1 1-e 1-e 0+e],c3);plot([0 1 1 0 0],[0 0 1 1 0]);disp('Mux');
  dotprod{1..30} (30 alike) : neural/Weight Functions/dotprod
  "iz{1,1}" : Outport
      mask Display: e = 0.06;c1 = [120 230 180]/255;c2 = ([120 230 180]+0)/(256+128);c3 = ([120 230 180]+128)/(256+128);patch([0 1 1 0],[0 0 1 1],c1);patch([0 1 1 1-e 1-e 0+e],[0 0 1 1-e 0+e 0+e],c2);patch([0 0 1 1-e 0+e 0+e],[0 1 1 1-e 1-e 0+e],c3);plot([0 1 1 0 0],[0 0 1 1 0]);
  wires:
  "IW{1,1}(1,:)'"/1 -> dotprod1/1
  "pd{1,1}"/1 -> dotprod1/2, dotprod2/2, dotprod3/2, dotprod4/2, dotprod5/2, dotprod6/2, dotprod7/2, dotprod8/2, dotprod9/2, dotprod10/2, dotprod11/2, dotprod12/2, dotprod13/2, dotprod14/2, dotprod15/2, dotprod16/2, dotprod17/2, dotprod18/2, dotprod19/2, dotprod20/2, dotprod21/2, dotprod22/2, dotprod23/2, dotprod24/2, dotprod25/2, dotprod26/2, dotprod27/2, dotprod28/2, dotprod29/2, dotprod30/2
  dotprod1/1 -> Mux/1
  "IW{1,1}(2,:)'"/1 -> dotprod2/1
  dotprod2/1 -> Mux/2
  "IW{1,1}(3,:)'"/1 -> dotprod3/1
  dotprod3/1 -> Mux/3
  "IW{1,1}(4,:)'"/1 -> dotprod4/1
  dotprod4/1 -> Mux/4
  "IW{1,1}(5,:)'"/1 -> dotprod5/1
  dotprod5/1 -> Mux/5
  "IW{1,1}(6,:)'"/1 -> dotprod6/1
  dotprod6/1 -> Mux/6
  "IW{1,1}(7,:)'"/1 -> dotprod7/1
  dotprod7/1 -> Mux/7
  "IW{1,1}(8,:)'"/1 -> dotprod8/1
  dotprod8/1 -> Mux/8
  "IW{1,1}(9,:)'"/1 -> dotprod9/1
  dotprod9/1 -> Mux/9
  "IW{1,1}(10,:)'"/1 -> dotprod10/1
  dotprod10/1 -> Mux/10
  "IW{1,1}(11,:)'"/1 -> dotprod11/1
  dotprod11/1 -> Mux/11
  "IW{1,1}(12,:)'"/1 -> dotprod12/1
  dotprod12/1 -> Mux/12
  "IW{1,1}(13,:)'"/1 -> dotprod13/1
  dotprod13/1 -> Mux/13
  "IW{1,1}(14,:)'"/1 -> dotprod14/1
  dotprod14/1 -> Mux/14
  "IW{1,1}(15,:)'"/1 -> dotprod15/1
  dotprod15/1 -> Mux/15
  "IW{1,1}(16,:)'"/1 -> dotprod16/1
  dotprod16/1 -> Mux/16
  "IW{1,1}(17,:)'"/1 -> dotprod17/1
  dotprod17/1 -> Mux/17
  "IW{1,1}(18,:)'"/1 -> dotprod18/1
  dotprod18/1 -> Mux/18
  "IW{1,1}(19,:)'"/1 -> dotprod19/1
  dotprod19/1 -> Mux/19
  "IW{1,1}(20,:)'"/1 -> dotprod20/1
  dotprod20/1 -> Mux/20
  "IW{1,1}(21,:)'"/1 -> dotprod21/1
  dotprod21/1 -> Mux/21
  "IW{1,1}(22,:)'"/1 -> dotprod22/1
  dotprod22/1 -> Mux/22
  "IW{1,1}(23,:)'"/1 -> dotprod23/1
  dotprod23/1 -> Mux/23
  "IW{1,1}(24,:)'"/1 -> dotprod24/1
  dotprod24/1 -> Mux/24
  "IW{1,1}(25,:)'"/1 -> dotprod25/1
  dotprod25/1 -> Mux/25
  "IW{1,1}(26,:)'"/1 -> dotprod26/1
  dotprod26/1 -> Mux/26
  "IW{1,1}(27,:)'"/1 -> dotprod27/1
  dotprod27/1 -> Mux/27
  "IW{1,1}(28,:)'"/1 -> dotprod28/1
  dotprod28/1 -> Mux/28
  "IW{1,1}(29,:)'"/1 -> dotprod29/1
  dotprod29/1 -> Mux/29
  "IW{1,1}(30,:)'"/1 -> dotprod30/1
  dotprod30/1 -> Mux/30
  Mux/1 -> "iz{1,1}"/1

== system e4_tank_reactor_no_error_dyn/NN_cex_1/Layer 2/Delays 1 ==
  "p{2}" : Inport  PortDimensions=30
      mask Display: e = 0.06;c1 = [120 230 180]/255;c2 = ([120 230 180]+0)/(256+128);c3 = ([120 230 180]+128)/(256+128);patch([0 1 1 0],[0 0 1 1],c1);patch([0 1 1 1-e 1-e 0+e],[0 0 1 1-e 0+e 0+e],c2);patch([0 0 1 1-e 0+e 0+e],[0 1 1 1-e 1-e 0+e],c3);plot([0 1 1 0 0],[0 0 1 1 0]);
  mux : Mux  Inputs=1
      mask Display: e = 0.06;c1 = [120 150 230]/255;c2 = ([120 150 230]+0)/383;c3 = ([120 150 230]+128)/383;patch([0 1 1 0],[0 0 1 1],c1);patch([0 1 1 1-e 1-e 0+e],[0 0 1 1-e 0+e 0+e],c2);patch([0 0 1 1-e 0+e 0+e],[0 1 1 1-e 1-e 0+e],c3);plot([0 1 1 0 0],[0 0 1 1 0]);disp('Mux')
  "pd{2,1}" : Outport
      mask Display: e = 0.06;c1 = [120 230 180]/255;c2 = ([120 230 180]+0)/(256+128);c3 = ([120 230 180]+128)/(256+128);patch([0 1 1 0],[0 0 1 1],c1);patch([0 1 1 1-e 1-e 0+e],[0 0 1 1-e 0+e 0+e],c2);patch([0 0 1 1-e 0+e 0+e],[0 1 1 1-e 1-e 0+e],c3);plot([0 1 1 0 0],[0 0 1 1 0]);
  wires:
  "p{2}"/1 -> mux/1
  mux/1 -> "pd{2,1}"/1
